simulink model "LinearMod"  (R2019b)
settings: Solver=VariableStepAuto  StartTime=0.0  StopTime=100  FixedStep=10e-3  RelTol=1e-3
values from neighbouring files (symbols this model uses):
  am1 = -1.3205    [discrete1.m]    (also in discrete2.m; dstr_demo.m; istr.m)
  am2 = 0.4966    [discrete1.m]    (also in discrete2.m; dstr_demo.m; istr.m)
  bm0 = 0.1761    [discrete1.m]    (also in discrete2.m; dstr_demo.m; istr.m)
  fs = -1    [discrete1.m]    (also in discrete2.m; istr.m)
  lambda_1 = 0.95    [discrete1.m]    (also in discrete2.m = 0.9; istr.m = 0.5)
  Pphi_0 = 100*eye(4)    [discrete1.m]    (also in discrete2.m)
  teta_phi_0 = [-1.5 0.5 2 2]    [discrete1.m]    (also in discrete2.m = [-1 0.5 3 1])
settings Model: Creator=user  LastModifiedBy=user

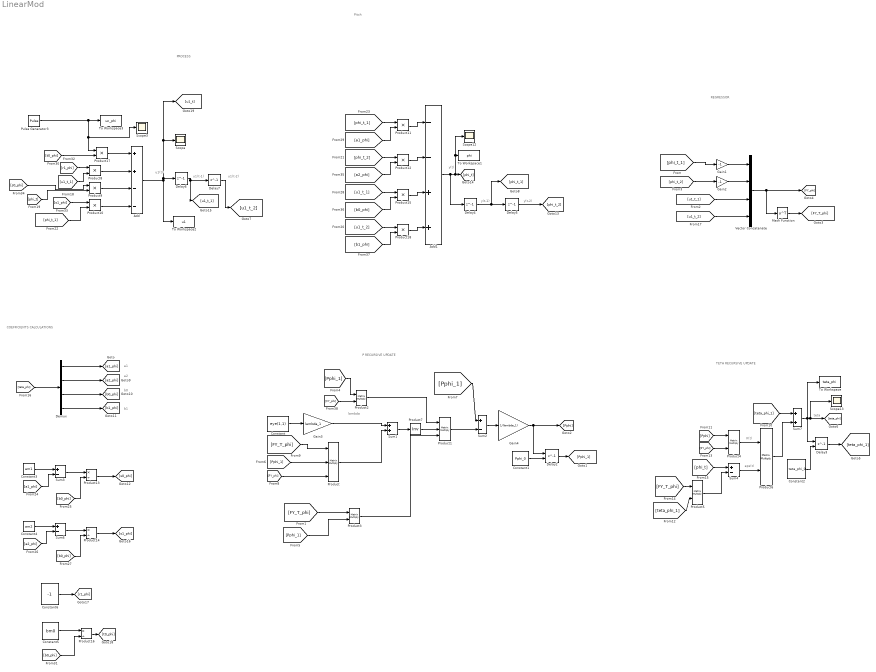
== system LinearMod ==
  note: Pitch
  note: COEFFICIENTS CALCULATIONS
  note: b1
  note: b0
  note: a2
  note: lambda
  note: K(t)
  note: eps(t)
  note: TETA RECURSIVE UPDATE
  note: PROCESS
  note: teta
  note: REGRESSOR
  note: y(t)
  note: a1
  note: y(t-1)
  note: P RECURSIVE UPDATE
  note: u1(t-2)
  note: u1(t-1)
  note: u1(t)
  note: y(t-2)
  Add : Sum  Inputs=++--
  Add1 : Sum  Inputs=--++
  Constant : Constant  Value=eye(1,1)
  Constant1 : Constant  Value=Pphi_0
  Constant2 : Constant  Value=teta_phi_0
  Constant3 : Constant  Value=am1
  Constant4 : Constant  Value=am2
  Constant5 : Constant  Value=bm0
  Constant6 : Constant  Value=-1
  Delay2 : Delay  DelayLength=1  InitialConditionSource=Input port  InitialCondition=0
      settings: InputPortMap=u0,p4
  Delay3 : Delay  DelayLength=1  InitialConditionSource=Input port  InitialCondition=0
      settings: InputPortMap=u0,p4
  Delay{4..7} (4 alike) : Delay  DelayLength=1  InitialCondition=0
  Demux : Demux
  Gain1 : Gain  Gain=-1
  Gain2 : Gain  Gain=-1
  Gain3 : Gain  Gain=lambda_1
  Gain4 : Gain  Gain=1/(lambda_1)
  Math Function : Math  Operator=transpose  SaturateOnIntegerOverflow=on
  Product : Product  Inputs=3  Multiplication=Matrix(*)
  Product1 : Product  Inputs=3  Multiplication=Matrix(*)
  Product{8..12,15,17..18} (8 alike) : Product
  Product13 : Product  Inputs=*/
  Product14 : Product  Inputs=*/
  Product16 : Product  Inputs=*/
  Product{2..6} (5 alike) : Product  Multiplication=Matrix(*)
  Product7 : Product  Inputs=/  Multiplication=Matrix(*)
  Pulse Generator3 : DiscretePulseGenerator  Period=30  PulseWidth=15  SampleTime=-1
  Scope{,3,12..13} (4 alike) : Scope
  Sum1 : Sum
  Sum{2..4,6} (4 alike) : Sum  Inputs=+-
  Sum7 : Sum
  To Workspace : ToWorkspace  VariableName=teta_phi  SampleTime=1/fs
  To Workspace1 : ToWorkspace  VariableName=phi  SampleTime=1/fs
  To Workspace2 : ToWorkspace  VariableName=u1  SampleTime=1/fs
  To Workspace3 : ToWorkspace  VariableName=uc_phi  SampleTime=1/fs
      settings: Save2DSignal=2-D array (concatenate along first dimension)
  Vector Concatenate : Concatenate  NumInputs=4
  wires:
  [u1_t_2] -> Vector Concatenate/4
  Product10/1 -> Add/4
  Math Function/1 -> [FY_T_phi]
  Demux/3 -> [b0_phi]
  [phi_t] -> Product9/2
  Product8/1 -> Add/2
  Product5/1 -> Sum4/2
  [Pphi] -> Product4/1
  Constant6/1 -> [r1_phi]
  Delay2/1 -> [Pphi_1]
  Gain4/1 -> [Pphi], Delay2/1
  [t0_phi] -> Product17/2
  Product13/1 -> [s0_phi]
  [s1_phi] -> Product10/1
  Pulse Generator3/1 -> Product17/1, Scope3/1, To Workspace3/1
  [phi_t_1] -> Gain1/1
  [a2_phi] -> Sum6/2
  Sum1/1 -> Product7/1
  [s0_phi] -> Product9/1
  Sum2/1 -> Gain4/1
  [u1_t_1] -> Product8/2
  Product9/1 -> Add/3
  Delay4/1 -> [phi_t_1], Delay5/1
  Delay6/1 -> Delay7/1, [u1_t_1]
  [Pphi_1] -> Product2/1
  Constant/1 -> Gain3/1
  Product17/1 -> Add/1
  Sum7/1 -> To Workspace/1, Scope13/1, [teta_phi], Delay3/1
  [phi_t_1] -> Product10/2
  Gain1/1 -> Vector Concatenate/1
  [b0_phi] -> Product14/2
  [FY_T_phi] -> Product/1
  Constant4/1 -> Sum6/1
  Product/1 -> Sum1/2
  Product1/1 -> Sum2/2
  Sum4/1 -> Product6/2
  [teta_phi_1] -> Product5/2
  Product4/1 -> Product6/1
  Demux/4 -> [b1_phi]
  Product14/1 -> [s1_phi]
  [Pphi_1] -> Sum2/1
  [r1_phi] -> Product8/1
  Delay5/1 -> [phi_t_2]
  [phi_t] -> Sum4/1
  Delay7/1 -> [u1_t_2]
  [FY_phi] -> Product/3
  Vector Concatenate/1 -> Math Function/1, [FY_phi]
  Demux/2 -> [a2_phi]
  [Pphi_1] -> Product3/2
  Gain3/1 -> Sum1/1
  [a1_phi] -> Sum3/2
  [teta_phi] -> Demux/1
  Gain2/1 -> Vector Concatenate/2
  [phi_t_2] -> Gain2/1
  Constant3/1 -> Sum3/1
  [Pphi_1] -> Product/2
  [b0_phi] -> Product13/2
  [FY_phi] -> Product4/2
  Constant5/1 -> Product16/1
  Demux/1 -> [a1_phi]
  [FY_T_phi] -> Product5/1
  Delay3/1 -> [teta_phi_1]
  Product3/1 -> Product1/3
  Add/1 -> [u1_t], Scope/1, Delay6/1, To Workspace2/1
  Product2/1 -> Product1/1
  [FY_T_phi] -> Product3/1
  Constant1/1 -> Delay2/2
  [teta_phi_1] -> Sum7/1
  [u1_t_1] -> Vector Concatenate/3
  Sum6/1 -> Product14/1
  [b0_phi] -> Product16/2
  Product16/1 -> [t0_phi]
  Sum3/1 -> Product13/1
  Product6/1 -> Sum7/2
  Product7/1 -> Product1/2
  Constant2/1 -> Delay3/2
  [phi_t_1] -> Product11/1
  Product11/1 -> Add1/1
  [a1_phi] -> Product11/2
  [a2_phi] -> Product12/2
  [phi_t_2] -> Product12/1
  Product12/1 -> Add1/2
  [b0_phi] -> Product15/2
  [u1_t_1] -> Product15/1
  Product15/1 -> Add1/3
  [b1_phi] -> Product18/2
  [u1_t_2] -> Product18/1
  Product18/1 -> Add1/4
  Add1/1 -> Delay4/1, Scope12/1, To Workspace1/1, [phi_t]
  [FY_phi] -> Product2/2
